simulink model "DynMdlSilver_20171112_1524"  (R2016b)
settings: Solver=VariableStepAuto  StartTime=0.0  StopTime=10.0  RelTol=1e-3
libraries: TM_DynamicModel_Library x117
settings Model: Creator=vpadmaj  LastModifiedBy=vpadmaj

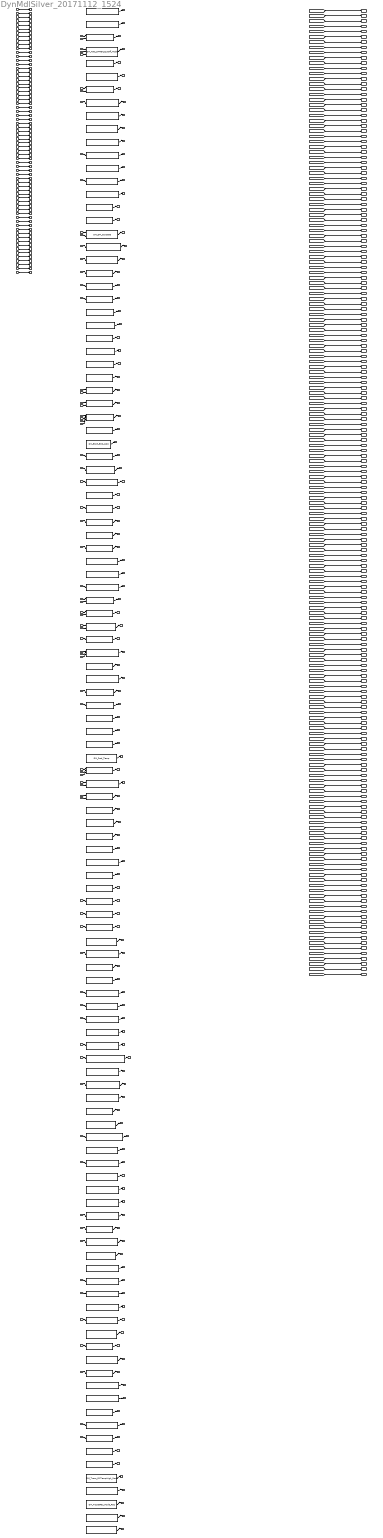
== system DynMdlSilver_20171112_1524 ==
  AAP : Inport
  AAT : Inport  Port=2
  AC_ShutterOpen_Req : Inport  Port=3
  AGB_WaterLevel : Inport  Port=4
  APP : Inport  Port=5
  AirFilOutP_P : Inport  Port=6
  AirFilOutTp_Tp : Inport  Port=7
  AmbAirP_P : Inport  Port=8
  AmbAirTp_Tp : Inport  Port=9
  Bat_Volt : Inport  Port=10
  Bms48_Cur : Inport  Port=11
  Bms48_Tp : Inport  Port=12
  Bms48_Volt : Inport  Port=13
  CacCooltTp_Tp : Inport  Port=14
  CacInTp_Tp : Inport  Port=15
  CacOutTp_Tp : Inport  Port=16
  ClpmpBms_ElecCurrAct : Inport  Port=17
  Dcdc1_CurHvDc : Inport  Port=18
  ECT : Inport  Port=19
  EIS_IgnSwState : Inport  Port=20
  EM2_Curr : Inport  Port=21
  EM2_InvrtTemp : Inport  Port=22
  EM2_Spd : Inport  Port=23
  EM2_Trq : Inport  Port=24
  EM2_TrqPlaus : Inport  Port=25
  EM2_Volt : Inport  Port=26
  ESOC_SOC : Inport  Port=27
  Eac_CurHvDc : Inport  Port=28
  Eac_VoltHvDc : Inport  Port=29
  Em01_CurHvDc : Inport  Port=30
  Em01_TpCooltOutInv : Inport  Port=31
  Em01_VoltHvDc : Inport  Port=32
  Emmo_VoltLinkPN48 : Inport  Port=33
  EngClpmp_FlgOnReq : Inport  Port=34
  EngCoolTp_Tp : Inport  Port=35
  EngCoolTp_TpMdl : Inport  Port=36
  EngOilP_P : Inport  Port=37
  EngOilTp_Tp : Inport  Port=38
  Eng_Fuel_Mass_Flow_Calc : Inport  Port=39
  Eng_Spd : Inport  Port=40
  Eng_Trq : Inport  Port=41
  Eng_Trq_Ind : Inport  Port=42
  ExtAir_Temp_Raw : Inport  Port=43
  Fu_Mp1 : Inport  Port=44
  Gear_State : Inport  Port=45
  IAT : Inport  Port=46
  IMAT : Inport  Port=47
  IntkAir_Temp : Inport  Port=48
  IntkVlvInP_P : Inport  Port=49
  LIN_BpShttrPosReq : Inport  Port=50
  LIN_CF_Spd_Req : Inport  Port=51
  LIN_CP_CACTransSpd_Req : Inport  Port=52
  LIN_RSV_CACTransPos_State : Inport  Port=53
  LIN_ShttrPosReq : Inport  Port=54
  MAF : Inport  Port=55
  Pnct48_DcdcCnvrTemp : Inport  Port=56
  Pnct48_PwrPackCoolOutTemp : Inport  Port=57
  TCM_Oil_Temp : Inport  Port=58
  ThrOutPSnsr_P : Inport  Port=59
  TmBmsCcr_SnsrTp : Inport  Port=60
  TmLtCcr_SnsrTpAct : Inport  Port=61
  TmPmp_EngClpmpLinReqPwm : Inport  Port=62
  Tm_BmsClpmpNReq : Inport  Port=63
  TrbInTp_Tp : Inport  Port=64
  VehMass_Wght_Pred : Inport  Port=65
  Veh_Spd : Inport  Port=66
  n_Eng : Inport  Port=67
  tp_ExhAtExhMnfld : Inport  Port=68
  DM_ACSwOff_Mode : TM_DynamicModel_Library/DM_ACSwOff_Mode
  DM_AC_HtrVlv_Front_Req : TM_DynamicModel_Library/DM_AC_HtrVlv_Front_Req
  DM_AGC_ASSStop_Mode : TM_DynamicModel_Library/DM_AGC_ASSStop_Mode
  DM_AGC_DTREngCutOff_Mode : TM_DynamicModel_Library/DM_AGC_DTREngCutOff_Mode
  DM_AGKInit_Mode : TM_DynamicModel_Library/DM_AGKInit_Mode
  DM_AT2_Mode : TM_DynamicModel_Library/DM_AT2_Mode
  DM_AdapAltitudeTempCorr_Coef : TM_DynamicModel_Library/DM_AdapAltitudeTempCorr_Coef
  DM_AdapAltitude_Coef : TM_DynamicModel_Library/DM_AdapAltitude_Coef
  DM_BMS_Batt_Temp : TM_DynamicModel_Library/DM_BMS_Batt_Temp
  DM_Bat_TotDchaProtnSwtSt : TM_DynamicModel_Library/DM_Bat_TotDchaProtnSwtSt
  DM_ChilExpVlv_RunSt : TM_DynamicModel_Library/DM_ChilExpVlv_RunSt
  DM_ClpmpBms_ElecRpmTrgtAct : TM_DynamicModel_Library/DM_ClpmpBms_ElecRpmTrgtAct
  DM_ClpmpBms_ElecTempAct : TM_DynamicModel_Library/DM_ClpmpBms_ElecTempAct
  DM_ClpmpBms_NAct : TM_DynamicModel_Library/DM_ClpmpBms_NAct
  DM_Cmpr1OutP_P : TM_DynamicModel_Library/DM_Cmpr1OutP_P
  DM_DCDC1_CoolTemp : TM_DynamicModel_Library/DM_DCDC1_CoolTemp
  DM_DCDC1_Temp : TM_DynamicModel_Library/DM_DCDC1_Temp
  DM_DFI_OprState : TM_DynamicModel_Library/DM_DFI_OprState
  DM_DFSO_Mode : TM_DynamicModel_Library/DM_DFSO_Mode
  DM_Dspl_EngShutOff_Time : TM_DynamicModel_Library/DM_Dspl_EngShutOff_Time
  DM_EACHV_Energy_Req : TM_DynamicModel_Library/DM_EACHV_Energy_Req
  DM_EACHV_SwClosed : TM_DynamicModel_Library/DM_EACHV_SwClosed
  DM_EACHV_SwOpen : TM_DynamicModel_Library/DM_EACHV_SwOpen
  DM_EATX_State : TM_DynamicModel_Library/DM_EATX_State
  DM_ECF_Pwr_Req : TM_DynamicModel_Library/DM_ECF_Pwr_Req
  DM_ECOMP_EAC_CompOn_Req : TM_DynamicModel_Library/DM_ECOMP_EAC_CompOn_Req
  DM_ECU_Temp : TM_DynamicModel_Library/DM_ECU_Temp
  DM_EFB_HV_Ready_Mode : TM_DynamicModel_Library/DM_EFB_HV_Ready_Mode
  DM_EM2_Cool_Req : TM_DynamicModel_Library/DM_EM2_Cool_Req
  DM_EM2_StMachn_State : TM_DynamicModel_Library/DM_EM2_StMachn_State
  DM_EM2_State_Req : TM_DynamicModel_Library/DM_EM2_State_Req
  DM_EM2_Temp : TM_DynamicModel_Library/DM_EM2_Temp
  DM_EOBC_Energy_Req : TM_DynamicModel_Library/DM_EOBC_Energy_Req
  DM_ESIG_BMS_SOC : TM_DynamicModel_Library/DM_ESIG_BMS_SOC
  DM_ESIG_BMS_Switch_State : TM_DynamicModel_Library/DM_ESIG_BMS_Switch_State
  DM_ESIG_Dspl_EngShutOff_Time : TM_DynamicModel_Library/DM_ESIG_Dspl_EngShutOff_Time
  DM_Ebtm_FlgHvBatChilCoolReq : TM_DynamicModel_Library/DM_Ebtm_FlgHvBatChilCoolReq
  DM_Ecobc_FlgBatHeatgReq : TM_DynamicModel_Library/DM_Ecobc_FlgBatHeatgReq
  DM_Ecu_St : TM_DynamicModel_Library/DM_Ecu_St
  DM_Ecu_StBusReq : TM_DynamicModel_Library/DM_Ecu_StBusReq
  DM_Efb_FlgHvRdyModPlaus : TM_DynamicModel_Library/DM_Efb_FlgHvRdyModPlaus
  DM_Em_PhaAcCur : TM_DynamicModel_Library/DM_Em_PhaAcCur
  DM_Emm_FlgNetSndrEna : TM_DynamicModel_Library/DM_Emm_FlgNetSndrEna
  DM_EngClpmp_PercPwrReq : TM_DynamicModel_Library/DM_EngClpmp_PercPwrReq
  DM_Eng_Actl_OpMode : TM_DynamicModel_Library/DM_Eng_Actl_OpMode
  DM_Eng_Cyc_Time : TM_DynamicModel_Library/DM_Eng_Cyc_Time
  DM_Eng_RelLoad : TM_DynamicModel_Library/DM_Eng_RelLoad
  DM_Eng_RelLoad_Req : TM_DynamicModel_Library/DM_Eng_RelLoad_Req
  DM_Eng_Run_Mode : TM_DynamicModel_Library/DM_Eng_Run_Mode
  DM_Eng_State_Actl : TM_DynamicModel_Library/DM_Eng_State_Actl
  DM_Eprec_FlgPreCdngAcvMod : TM_DynamicModel_Library/DM_Eprec_FlgPreCdngAcvMod
  DM_Err_ECT_low : TM_DynamicModel_Library/DM_Err_ECT_low
  DM_Esig_BmsTpMax : TM_DynamicModel_Library/DM_Esig_BmsTpMax
  DM_Esig_BmsTpMin : TM_DynamicModel_Library/DM_Esig_BmsTpMin
  DM_Esig_BmsTpTar : TM_DynamicModel_Library/DM_Esig_BmsTpTar
  DM_FRT_Sens : TM_DynamicModel_Library/DM_FRT_Sens
  DM_FirstStrt_Mode : TM_DynamicModel_Library/DM_FirstStrt_Mode
  DM_Fuel_Temp : TM_DynamicModel_Library/DM_Fuel_Temp
  DM_HDC_HybAggr_State : TM_DynamicModel_Library/DM_HDC_HybAggr_State
  DM_HDC_HybSync_State : TM_DynamicModel_Library/DM_HDC_HybSync_State
  DM_HDC_PTReady_Mode : TM_DynamicModel_Library/DM_HDC_PTReady_Mode
  DM_HVAC_CoolVlv_Rq : TM_DynamicModel_Library/DM_HVAC_CoolVlv_Rq
  DM_Hepm_PwrMax48VEcm : TM_DynamicModel_Library/DM_Hepm_PwrMax48VEcm
  DM_Hpmc_StPlgnOpmdDispd : TM_DynamicModel_Library/DM_Hpmc_StPlgnOpmdDispd
  DM_HvacChil_ExpVlvPosnReq : TM_DynamicModel_Library/DM_HvacChil_ExpVlvPosnReq
  DM_Hvac_StDefrstAcv : TM_DynamicModel_Library/DM_Hvac_StDefrstAcv
  DM_IC_Knk_Red_Avg : TM_DynamicModel_Library/DM_IC_Knk_Red_Avg
  DM_IC_Knk_Red_Avg_Actv : TM_DynamicModel_Library/DM_IC_Knk_Red_Avg_Actv
  DM_Idle_Mode_Req : TM_DynamicModel_Library/DM_Idle_Mode_Req
  DM_IgnSwStrtr_Mode : TM_DynamicModel_Library/DM_IgnSwStrtr_Mode
  DM_Ign_Mode : TM_DynamicModel_Library/DM_Ign_Mode
  DM_Injr_Tp : TM_DynamicModel_Library/DM_Injr_Tp
  DM_K15 : TM_DynamicModel_Library/DM_K15
  DM_LIN_BpShttrGrOvrTemp105_Mode : TM_DynamicModel_Library/DM_LIN_BpShttrGrOvrTemp105_Mode
  DM_LIN_BpShttrGrOvrTemp_Mode : TM_DynamicModel_Library/DM_LIN_BpShttrGrOvrTemp_Mode
  DM_LIN_BpShttrPosAct_Val : TM_DynamicModel_Library/DM_LIN_BpShttrPosAct_Val
  DM_LIN_CF_SpdAvg : TM_DynamicModel_Library/DM_LIN_CF_SpdAvg
  DM_LIN_CP_CAC2TransActlSpd : TM_DynamicModel_Library/DM_LIN_CP_CAC2TransActlSpd
  DM_LIN_CP_CAC2TransTp : TM_DynamicModel_Library/DM_LIN_CP_CAC2TransTp
  DM_LIN_CP_CACTransActlSpd : TM_DynamicModel_Library/DM_LIN_CP_CACTransActlSpd
  DM_LIN_CP_CACTransTgtSpd : TM_DynamicModel_Library/DM_LIN_CP_CACTransTgtSpd
  DM_LIN_CP_CACTransTp : TM_DynamicModel_Library/DM_LIN_CP_CACTransTp
  DM_LIN_CP_ECP4TransActlSpd : TM_DynamicModel_Library/DM_LIN_CP_ECP4TransActlSpd
  DM_LIN_CP_ECP4TransTp : TM_DynamicModel_Library/DM_LIN_CP_ECP4TransTp
  DM_LIN_CP_ECP4TransVoltClass : TM_DynamicModel_Library/DM_LIN_CP_ECP4TransVoltClass
  DM_LIN_CP_ECP4TransVoltStat : TM_DynamicModel_Library/DM_LIN_CP_ECP4TransVoltStat
  DM_LIN_RSV1_CACTransPos_State : TM_DynamicModel_Library/DM_LIN_RSV1_CACTransPos_State
  DM_LIN_RSV_CACTransMove_State : TM_DynamicModel_Library/DM_LIN_RSV_CACTransMove_State
  DM_LIN_ShttrPosAct_Val : TM_DynamicModel_Library/DM_LIN_ShttrPosAct_Val
  DM_LIN_ShttrPosMove_State : TM_DynamicModel_Library/DM_LIN_ShttrPosMove_State
  DM_MTX_Mode : TM_DynamicModel_Library/DM_MTX_Mode
  DM_Net_EBoost_CurrCons : TM_DynamicModel_Library/DM_Net_EBoost_CurrCons
  DM_Net_Eboost_PCB_Temp : TM_DynamicModel_Library/DM_Net_Eboost_PCB_Temp
  DM_Odo_Abs_HighRes : TM_DynamicModel_Library/DM_Odo_Abs_HighRes
  DM_Odo_Abs_Long : TM_DynamicModel_Library/DM_Odo_Abs_Long
  DM_Pnct48V_VoltMinThdShutDwnEcm : TM_DynamicModel_Library/DM_Pnct48V_VoltMinThdShutDwnEcm
  DM_Pnct48_HtCoolPwrRq : TM_DynamicModel_Library/DM_Pnct48_HtCoolPwrRq
  DM_Pnct48_PwrPackBatTempMax : TM_DynamicModel_Library/DM_Pnct48_PwrPackBatTempMax
  DM_Pnct48_PwrPackBatTempMin : TM_DynamicModel_Library/DM_Pnct48_PwrPackBatTempMin
  DM_RsvBms_PosnAct : TM_DynamicModel_Library/DM_RsvBms_PosnAct
  DM_RsvLoTpCcr_PosnAvlFlg : TM_DynamicModel_Library/DM_RsvLoTpCcr_PosnAvlFlg
  DM_ScrcmDos_THeatrPmpAftRunReq : TM_DynamicModel_Library/DM_ScrcmDos_THeatrPmpAftRunReq
  DM_TCC_Spd : TM_DynamicModel_Library/DM_TCC_Spd
  DM_Tc_FlgTpCrit : TM_DynamicModel_Library/DM_Tc_FlgTpCrit
  DM_TmBmsCcr_SnsrTpRaw : TM_DynamicModel_Library/DM_TmBmsCcr_SnsrTpRaw
  DM_TmBmsPSnsrChil_VoltRaw : TM_DynamicModel_Library/DM_TmBmsPSnsrChil_VoltRaw
  DM_TmBmsTpSnsrChil_ActVoltRaw : TM_DynamicModel_Library/DM_TmBmsTpSnsrChil_ActVoltRaw
  DM_TmGbOil_PredCtlAcvnFlg : TM_DynamicModel_Library/DM_TmGbOil_PredCtlAcvnFlg
  DM_TmLoTpCcr2_FillLvlVoltRaw : TM_DynamicModel_Library/DM_TmLoTpCcr2_FillLvlVoltRaw
  DM_TmLoTpCcr_SnsrTpRaw : TM_DynamicModel_Library/DM_TmLoTpCcr_SnsrTpRaw
  DM_TmPredHvBatCoolg_TpSpAcvFlg : TM_DynamicModel_Library/DM_TmPredHvBatCoolg_TpSpAcvFlg
  DM_TmPredQckwnsBatCoolt_BatTpSp : TM_DynamicModel_Library/DM_TmPredQckwnsBatCoolt_BatTpSp
  DM_Trans_OilTempHigh_Mode : TM_DynamicModel_Library/DM_Trans_OilTempHigh_Mode
  DM_TrqSetIgn_Mode_Req : TM_DynamicModel_Library/DM_TrqSetIgn_Mode_Req
  DM_TrqSetRes_Mode_Req : TM_DynamicModel_Library/DM_TrqSetRes_Mode_Req
  DM_ag_CamsftExhSp : TM_DynamicModel_Library/DM_ag_CamsftExhSp
  DM_ag_CamsftIntkSp : TM_DynamicModel_Library/DM_ag_CamsftIntkSp
  Dyn_AAP : Outport
  Dyn_AAT : Outport  Port=2
  Dyn_ACSwOff_Mode : Outport  Port=3
  Dyn_AC_HtrVlv_Front_Req : Outport  Port=4
  Dyn_AC_ShutterOpen_Req : Outport  Port=5
  Dyn_AGB_WaterLevel : Outport  Port=6
  Dyn_AGC_ASSStop_Mode : Outport  Port=7
  Dyn_AGC_DTREngCutOff_Mode : Outport  Port=8
  Dyn_AGKInit_Mode : Outport  Port=9
  Dyn_APP : Outport  Port=10
  Dyn_AT2_Mode : Outport  Port=11
  Dyn_AdapAltitudeTempCorr_Coef : Outport  Port=12
  Dyn_AdapAltitude_Coef : Outport  Port=13
  Dyn_AirFilOutP_P : Outport  Port=14
  Dyn_AirFilOutTp_Tp : Outport  Port=15
  Dyn_AmbAirP_P : Outport  Port=16
  Dyn_AmbAirTp_Tp : Outport  Port=17
  Dyn_BMS_Batt_Temp : Outport  Port=18
  Dyn_Bat_TotDchaProtnSwtSt : Outport  Port=19
  Dyn_Bat_Volt : Outport  Port=20
  Dyn_Bms48_Cur : Outport  Port=21
  Dyn_Bms48_Tp : Outport  Port=22
  Dyn_Bms48_Volt : Outport  Port=23
  Dyn_CacCooltTp_Tp : Outport  Port=24
  Dyn_CacInTp_Tp : Outport  Port=25
  Dyn_CacOutTp_Tp : Outport  Port=26
  Dyn_ChilExpVlv_RunSt : Outport  Port=27
  Dyn_ClpmpBms_ElecCurrAct : Outport  Port=28
  Dyn_ClpmpBms_ElecRpmTrgtAct : Outport  Port=29
  Dyn_ClpmpBms_ElecTempAct : Outport  Port=30
  Dyn_ClpmpBms_NAct : Outport  Port=31
  Dyn_Cmpr1OutP_P : Outport  Port=32
  Dyn_DCDC1_CoolTemp : Outport  Port=33
  Dyn_DCDC1_Temp : Outport  Port=34
  Dyn_DFI_OprState : Outport  Port=35
  Dyn_DFSO_Mode : Outport  Port=36
  Dyn_Dcdc1_CurHvDc : Outport  Port=37
  Dyn_Dspl_EngShutOff_Time : Outport  Port=38
  Dyn_EACHV_Energy_Req : Outport  Port=39
  Dyn_EACHV_SwClosed : Outport  Port=40
  Dyn_EACHV_SwOpen : Outport  Port=41
  Dyn_EATX_State : Outport  Port=42
  Dyn_ECF_Pwr_Req : Outport  Port=43
  Dyn_ECOMP_EAC_CompOn_Req : Outport  Port=44
  Dyn_ECT : Outport  Port=45
  Dyn_ECU_Temp : Outport  Port=46
  Dyn_EFB_HV_Ready_Mode : Outport  Port=47
  Dyn_EIS_IgnSwState : Outport  Port=48
  Dyn_EM2_Cool_Req : Outport  Port=49
  Dyn_EM2_Curr : Outport  Port=50
  Dyn_EM2_InvrtTemp : Outport  Port=51
  Dyn_EM2_Spd : Outport  Port=52
  Dyn_EM2_StMachn_State : Outport  Port=53
  Dyn_EM2_State_Req : Outport  Port=54
  Dyn_EM2_Temp : Outport  Port=55
  Dyn_EM2_Trq : Outport  Port=56
  Dyn_EM2_TrqPlaus : Outport  Port=57
  Dyn_EM2_Volt : Outport  Port=58
  Dyn_EOBC_Energy_Req : Outport  Port=59
  Dyn_ESIG_BMS_SOC : Outport  Port=60
  Dyn_ESIG_BMS_Switch_State : Outport  Port=61
  Dyn_ESIG_Dspl_EngShutOff_Time : Outport  Port=62
  Dyn_ESOC_SOC : Outport  Port=63
  Dyn_Eac_CurHvDc : Outport  Port=64
  Dyn_Eac_VoltHvDc : Outport  Port=65
  Dyn_Ebtm_FlgHvBatChilCoolReq : Outport  Port=66
  Dyn_Ecobc_FlgBatHeatgReq : Outport  Port=67
  Dyn_Ecu_St : Outport  Port=68
  Dyn_Ecu_StBusReq : Outport  Port=69
  Dyn_Efb_FlgHvRdyModPlaus : Outport  Port=70
  Dyn_Em01_CurHvDc : Outport  Port=71
  Dyn_Em01_TpCooltOutInv : Outport  Port=72
  Dyn_Em01_VoltHvDc : Outport  Port=73
  Dyn_Em_PhaAcCur : Outport  Port=74
  Dyn_Emm_FlgNetSndrEna : Outport  Port=75
  Dyn_Emmo_VoltLinkPN48 : Outport  Port=76
  Dyn_EngClpmp_FlgOnReq : Outport  Port=77
  Dyn_EngClpmp_PercPwrReq : Outport  Port=78
  Dyn_EngCoolTp_Tp : Outport  Port=79
  Dyn_EngCoolTp_TpMdl : Outport  Port=80
  Dyn_EngOilP_P : Outport  Port=81
  Dyn_EngOilTp_Tp : Outport  Port=82
  Dyn_Eng_Actl_OpMode : Outport  Port=83
  Dyn_Eng_Cyc_Time : Outport  Port=84
  Dyn_Eng_Fuel_Mass_Flow_Calc : Outport  Port=85
  Dyn_Eng_RelLoad : Outport  Port=86
  Dyn_Eng_RelLoad_Req : Outport  Port=87
  Dyn_Eng_Run_Mode : Outport  Port=88
  Dyn_Eng_Spd : Outport  Port=89
  Dyn_Eng_State_Actl : Outport  Port=90
  Dyn_Eng_Trq : Outport  Port=91
  Dyn_Eng_Trq_Ind : Outport  Port=92
  Dyn_Eprec_FlgPreCdngAcvMod : Outport  Port=93
  Dyn_Err_ECT_low : Outport  Port=94
  Dyn_Esig_BmsTpMax : Outport  Port=95
  Dyn_Esig_BmsTpMin : Outport  Port=96
  Dyn_Esig_BmsTpTar : Outport  Port=97
  Dyn_ExtAir_Temp_Raw : Outport  Port=98
  Dyn_FRT_Sens : Outport  Port=99
  Dyn_FirstStrt_Mode : Outport  Port=100
  Dyn_Fu_Mp1 : Outport  Port=101
  Dyn_Fuel_Temp : Outport  Port=102
  Dyn_Gear_State : Outport  Port=103
  Dyn_HDC_HybAggr_State : Outport  Port=104
  Dyn_HDC_HybSync_State : Outport  Port=105
  Dyn_HDC_PTReady_Mode : Outport  Port=106
  Dyn_HVAC_CoolVlv_Rq : Outport  Port=107
  Dyn_Hepm_PwrMax48VEcm : Outport  Port=108
  Dyn_Hpmc_StPlgnOpmdDispd : Outport  Port=109
  Dyn_HvacChil_ExpVlvPosnReq : Outport  Port=110
  Dyn_Hvac_StDefrstAcv : Outport  Port=111
  Dyn_IAT : Outport  Port=112
  Dyn_IC_Knk_Red_Avg : Outport  Port=113
  Dyn_IC_Knk_Red_Avg_Actv : Outport  Port=114
  Dyn_IMAT : Outport  Port=115
  Dyn_Idle_Mode_Req : Outport  Port=116
  Dyn_IgnSwStrtr_Mode : Outport  Port=117
  Dyn_Ign_Mode : Outport  Port=118
  Dyn_Injr_Tp : Outport  Port=119
  Dyn_IntkAir_Temp : Outport  Port=120
  Dyn_IntkVlvInP_P : Outport  Port=121
  Dyn_K15 : Outport  Port=122
  Dyn_LIN_BpShttrGrOvrTemp105_Mode : Outport  Port=123
  Dyn_LIN_BpShttrGrOvrTemp_Mode : Outport  Port=124
  Dyn_LIN_BpShttrPosAct_Val : Outport  Port=125
  Dyn_LIN_BpShttrPosReq : Outport  Port=126
  Dyn_LIN_CF_SpdAvg : Outport  Port=127
  Dyn_LIN_CF_Spd_Req : Outport  Port=128
  Dyn_LIN_CP_CAC2TransActlSpd : Outport  Port=129
  Dyn_LIN_CP_CAC2TransTp : Outport  Port=130
  Dyn_LIN_CP_CACTransActlSpd : Outport  Port=131
  Dyn_LIN_CP_CACTransSpd_Req : Outport  Port=132
  Dyn_LIN_CP_CACTransTgtSpd : Outport  Port=133
  Dyn_LIN_CP_CACTransTp : Outport  Port=134
  Dyn_LIN_CP_ECP4TransActlSpd : Outport  Port=135
  Dyn_LIN_CP_ECP4TransTp : Outport  Port=136
  Dyn_LIN_CP_ECP4TransVoltClass : Outport  Port=137
  Dyn_LIN_CP_ECP4TransVoltStat : Outport  Port=138
  Dyn_LIN_RSV1_CACTransPos_State : Outport  Port=139
  Dyn_LIN_RSV_CACTransMove_State : Outport  Port=140
  Dyn_LIN_RSV_CACTransPos_State : Outport  Port=141
  Dyn_LIN_ShttrPosAct_Val : Outport  Port=142
  Dyn_LIN_ShttrPosMove_State : Outport  Port=143
  Dyn_LIN_ShttrPosReq : Outport  Port=144
  Dyn_MAF : Outport  Port=145
  Dyn_MTX_Mode : Outport  Port=146
  Dyn_Net_EBoost_CurrCons : Outport  Port=147
  Dyn_Net_Eboost_PCB_Temp : Outport  Port=148
  Dyn_Odo_Abs_HighRes : Outport  Port=149
  Dyn_Odo_Abs_Long : Outport  Port=150
  Dyn_Pnct48V_VoltMinThdShutDwnEcm : Outport  Port=151
  Dyn_Pnct48_DcdcCnvrTemp : Outport  Port=152
  Dyn_Pnct48_HtCoolPwrRq : Outport  Port=153
  Dyn_Pnct48_PwrPackBatTempMax : Outport  Port=154
  Dyn_Pnct48_PwrPackBatTempMin : Outport  Port=155
  Dyn_Pnct48_PwrPackCoolOutTemp : Outport  Port=156
  Dyn_RsvBms_PosnAct : Outport  Port=157
  Dyn_RsvLoTpCcr_PosnAvlFlg : Outport  Port=158
  Dyn_ScrcmDos_THeatrPmpAftRunReq : Outport  Port=159
  Dyn_TCC_Spd : Outport  Port=160
  Dyn_TCM_Oil_Temp : Outport  Port=161
  Dyn_Tc_FlgTpCrit : Outport  Port=162
  Dyn_ThrOutPSnsr_P : Outport  Port=163
  Dyn_TmBmsCcr_SnsrTp : Outport  Port=164
  Dyn_TmBmsCcr_SnsrTpRaw : Outport  Port=165
  Dyn_TmBmsPSnsrChil_VoltRaw : Outport  Port=166
  Dyn_TmBmsTpSnsrChil_ActVoltRaw : Outport  Port=167
  Dyn_TmGbOil_PredCtlAcvnFlg : Outport  Port=168
  Dyn_TmLoTpCcr2_FillLvlVoltRaw : Outport  Port=169
  Dyn_TmLoTpCcr_SnsrTpRaw : Outport  Port=170
  Dyn_TmLtCcr_SnsrTpAct : Outport  Port=171
  Dyn_TmPmp_EngClpmpLinReqPwm : Outport  Port=172
  Dyn_TmPredHvBatCoolg_TpSpAcvFlg : Outport  Port=173
  Dyn_TmPredQckwnsBatCoolt_BatTpSp : Outport  Port=174
  Dyn_Tm_BmsClpmpNReq : Outport  Port=175
  Dyn_Trans_OilTempHigh_Mode : Outport  Port=176
  Dyn_TrbInTp_Tp : Outport  Port=177
  Dyn_TrqSetIgn_Mode_Req : Outport  Port=178
  Dyn_TrqSetRes_Mode_Req : Outport  Port=179
  Dyn_VehMass_Wght_Pred : Outport  Port=180
  Dyn_Veh_Spd : Outport  Port=181
  Dyn_ag_CamsftExhSp : Outport  Port=182
  Dyn_ag_CamsftIntkSp : Outport  Port=183
  Dyn_n_Eng : Outport  Port=184
  Dyn_tp_ExhAtExhMnfld : Outport  Port=185
  wires:
  DM_ACSwOff_Mode/1 -> [ACSwOff_Mode]
  DM_AC_HtrVlv_Front_Req/1 -> [AC_HtrVlv_Front_Req]
  [Eng_Spd] -> DM_AGC_ASSStop_Mode/1
  [Eng_Trq] -> DM_AGC_ASSStop_Mode/2
  DM_AGC_ASSStop_Mode/1 -> [AGC_ASSStop_Mode]
  [Eng_Trq] -> DM_AGC_DTREngCutOff_Mode/1
  [EIS_IgnSwState] -> DM_AGC_DTREngCutOff_Mode/2
  [Eng_Spd] -> DM_AGC_DTREngCutOff_Mode/3
  DM_AGC_DTREngCutOff_Mode/1 -> [AGC_DTREngCutOff_Mode]
  DM_AGKInit_Mode/1 -> [AGKInit_Mode]
  DM_AT2_Mode/1 -> [AT2_Mode]
  [AmbAirP_P] -> DM_AdapAltitudeTempCorr_Coef/1
  [IntkAir_Temp] -> DM_AdapAltitudeTempCorr_Coef/2
  DM_AdapAltitudeTempCorr_Coef/1 -> [AdapAltitudeTempCorr_Coef]
  [AmbAirP_P] -> DM_AdapAltitude_Coef/1
  DM_AdapAltitude_Coef/1 -> [AdapAltitude_Coef]
  DM_BMS_Batt_Temp/1 -> [BMS_Batt_Temp]
  DM_Bat_TotDchaProtnSwtSt/1 -> [Bat_TotDchaProtnSwtSt]
  DM_ChilExpVlv_RunSt/1 -> [ChilExpVlv_RunSt]
  [Tm_BmsClpmpNReq] -> DM_ClpmpBms_ElecRpmTrgtAct/1
  DM_ClpmpBms_ElecRpmTrgtAct/1 -> [ClpmpBms_ElecRpmTrgtAct]
  DM_ClpmpBms_ElecTempAct/1 -> [ClpmpBms_ElecTempAct]
  [Tm_BmsClpmpNReq] -> DM_ClpmpBms_NAct/1
  DM_ClpmpBms_NAct/1 -> [ClpmpBms_NAct]
  DM_Cmpr1OutP_P/1 -> [Cmpr1OutP_P]
  DM_DCDC1_CoolTemp/1 -> [DCDC1_CoolTemp]
  DM_DCDC1_Temp/1 -> [DCDC1_Temp]
  [MAF] -> DM_DFI_OprState/1
  [Eng_Fuel_Mass_Flow_Calc] -> DM_DFI_OprState/2
  DM_DFI_OprState/1 -> [DFI_OprState]
  [Veh_Spd] -> DM_DFSO_Mode/1
  DM_DFSO_Mode/1 -> [DFSO_Mode]
  [Eng_Spd] -> DM_Dspl_EngShutOff_Time/1
  DM_Dspl_EngShutOff_Time/1 -> [Dspl_EngShutOff_Time]
  [EIS_IgnSwState] -> DM_EACHV_Energy_Req/1
  DM_EACHV_Energy_Req/1 -> [EACHV_Energy_Req]
  [EIS_IgnSwState] -> DM_EACHV_SwClosed/1
  DM_EACHV_SwClosed/1 -> [EACHV_SwClosed]
  [EIS_IgnSwState] -> DM_EACHV_SwOpen/1
  DM_EACHV_SwOpen/1 -> [EACHV_SwOpen]
  DM_EATX_State/1 -> [EATX_State]
  DM_ECF_Pwr_Req/1 -> [ECF_Pwr_Req]
  DM_ECOMP_EAC_CompOn_Req/1 -> [ECOMP_EAC_CompOn_Req]
  DM_ECU_Temp/1 -> [ECU_Temp]
  DM_EFB_HV_Ready_Mode/1 -> [EFB_HV_Ready_Mode]
  DM_EM2_Cool_Req/1 -> [EM2_Cool_Req]
  [Eng_Spd] -> DM_EM2_StMachn_State/1
  [EIS_IgnSwState] -> DM_EM2_StMachn_State/2
  DM_EM2_StMachn_State/1 -> [EM2_StMachn_State]
  [Eng_Spd] -> DM_EM2_State_Req/1
  [Gear_State] -> DM_EM2_State_Req/2
  DM_EM2_State_Req/1 -> [EM2_State_Req]
  [EM2_Volt] -> DM_EM2_Temp/1
  [EM2_Curr] -> DM_EM2_Temp/2
  [EM2_Trq] -> DM_EM2_Temp/3
  [EM2_Spd] -> DM_EM2_Temp/4
  DM_EM2_Temp/1 -> [EM2_Temp]
  DM_EOBC_Energy_Req/1 -> [EOBC_Energy_Req]
  DM_ESIG_BMS_SOC/1 -> [ESIG_BMS_SOC]
  [EIS_IgnSwState] -> DM_ESIG_BMS_Switch_State/1
  DM_ESIG_BMS_Switch_State/1 -> [ESIG_BMS_Switch_State]
  [Eng_Spd] -> DM_ESIG_Dspl_EngShutOff_Time/1
  DM_ESIG_Dspl_EngShutOff_Time/1 -> [ESIG_Dspl_EngShutOff_Time]
  [Bms48_Tp] -> DM_Ebtm_FlgHvBatChilCoolReq/1
  DM_Ebtm_FlgHvBatChilCoolReq/1 -> [Ebtm_FlgHvBatChilCoolReq]
  DM_Ecobc_FlgBatHeatgReq/1 -> [Ecobc_FlgBatHeatgReq]
  [EIS_IgnSwState] -> DM_Ecu_St/1
  DM_Ecu_St/1 -> [Ecu_St]
  [EIS_IgnSwState] -> DM_Ecu_StBusReq/1
  DM_Ecu_StBusReq/1 -> [Ecu_StBusReq]
  DM_Efb_FlgHvRdyModPlaus/1 -> [Efb_FlgHvRdyModPlaus]
  [EM2_Trq] -> DM_Em_PhaAcCur/1
  DM_Em_PhaAcCur/1 -> [Em_PhaAcCur]
  DM_Emm_FlgNetSndrEna/1 -> [Emm_FlgNetSndrEna]
  DM_EngClpmp_PercPwrReq/1 -> [EngClpmp_PercPwrReq]
  [Eng_State_Actl] -> DM_Eng_Actl_OpMode/1
  DM_Eng_Actl_OpMode/1 -> [Eng_Actl_OpMode]
  [Eng_Spd] -> DM_Eng_Cyc_Time/1
  [EIS_IgnSwState] -> DM_Eng_Cyc_Time/2
  DM_Eng_Cyc_Time/1 -> [Eng_Cyc_Time]
  [MAF] -> DM_Eng_RelLoad/1
  [Eng_Spd] -> DM_Eng_RelLoad/2
  DM_Eng_RelLoad/1 -> [Eng_RelLoad]
  [MAF] -> DM_Eng_RelLoad_Req/1
  [Eng_Spd] -> DM_Eng_RelLoad_Req/2
  DM_Eng_RelLoad_Req/1 -> [Eng_RelLoad_Req]
  [Eng_Spd] -> DM_Eng_Run_Mode/1
  DM_Eng_Run_Mode/1 -> [Eng_Run_Mode]
  [K15] -> DM_Eng_State_Actl/1
  [Eng_Spd] -> DM_Eng_State_Actl/2
  [AGC_ASSStop_Mode] -> DM_Eng_State_Actl/3
  DM_Eng_State_Actl/1 -> [Eng_State_Actl]
  DM_Eprec_FlgPreCdngAcvMod/1 -> [Eprec_FlgPreCdngAcvMod]
  DM_Err_ECT_low/1 -> [Err_ECT_low]
  [Bms48_Tp] -> DM_Esig_BmsTpMax/1
  DM_Esig_BmsTpMax/1 -> [Esig_BmsTpMax]
  [Bms48_Tp] -> DM_Esig_BmsTpMin/1
  DM_Esig_BmsTpMin/1 -> [Esig_BmsTpMin]
  DM_Esig_BmsTpTar/1 -> [Esig_BmsTpTar]
  DM_FRT_Sens/1 -> [FRT_Sens]
  DM_FirstStrt_Mode/1 -> [FirstStrt_Mode]
  DM_Fuel_Temp/1 -> [Fuel_Temp]
  [EIS_IgnSwState] -> DM_HDC_HybAggr_State/1
  [Eng_Spd] -> DM_HDC_HybAggr_State/2
  [Gear_State] -> DM_HDC_HybAggr_State/3
  DM_HDC_HybAggr_State/1 -> [HDC_HybAggr_State]
  [Eng_Spd] -> DM_HDC_HybSync_State/1
  [Eng_Trq] -> DM_HDC_HybSync_State/2
  DM_HDC_HybSync_State/1 -> [HDC_HybSync_State]
  [Eng_Spd] -> DM_HDC_PTReady_Mode/1
  [EIS_IgnSwState] -> DM_HDC_PTReady_Mode/2
  DM_HDC_PTReady_Mode/1 -> [HDC_PTReady_Mode]
  DM_HVAC_CoolVlv_Rq/1 -> [HVAC_CoolVlv_Rq]
  DM_Hepm_PwrMax48VEcm/1 -> [Hepm_PwrMax48VEcm]
  DM_Hpmc_StPlgnOpmdDispd/1 -> [Hpmc_StPlgnOpmdDispd]
  DM_HvacChil_ExpVlvPosnReq/1 -> [HvacChil_ExpVlvPosnReq]
  DM_Hvac_StDefrstAcv/1 -> [Hvac_StDefrstAcv]
  DM_IC_Knk_Red_Avg/1 -> [IC_Knk_Red_Avg]
  DM_IC_Knk_Red_Avg_Actv/1 -> [IC_Knk_Red_Avg_Actv]
  [APP] -> DM_Idle_Mode_Req/1
  DM_Idle_Mode_Req/1 -> [Idle_Mode_Req]
  [EIS_IgnSwState] -> DM_IgnSwStrtr_Mode/1
  DM_IgnSwStrtr_Mode/1 -> [IgnSwStrtr_Mode]
  [EIS_IgnSwState] -> DM_Ign_Mode/1
  DM_Ign_Mode/1 -> [Ign_Mode]
  DM_Injr_Tp/1 -> [Injr_Tp]
  [EIS_IgnSwState] -> DM_K15/1
  DM_K15/1 -> [K15]
  DM_LIN_BpShttrGrOvrTemp105_Mode/1 -> [LIN_BpShttrGrOvrTemp105_Mode]
  DM_LIN_BpShttrGrOvrTemp_Mode/1 -> [LIN_BpShttrGrOvrTemp_Mode]
  [LIN_BpShttrPosReq] -> DM_LIN_BpShttrPosAct_Val/1
  DM_LIN_BpShttrPosAct_Val/1 -> [LIN_BpShttrPosAct_Val]
  [LIN_CF_Spd_Req] -> DM_LIN_CF_SpdAvg/1
  DM_LIN_CF_SpdAvg/1 -> [LIN_CF_SpdAvg]
  [Tm_BmsClpmpNReq] -> DM_LIN_CP_CAC2TransActlSpd/1
  DM_LIN_CP_CAC2TransActlSpd/1 -> [LIN_CP_CAC2TransActlSpd]
  DM_LIN_CP_CAC2TransTp/1 -> [LIN_CP_CAC2TransTp]
  [LIN_CP_CACTransSpd_Req] -> DM_LIN_CP_CACTransActlSpd/1
  DM_LIN_CP_CACTransActlSpd/1 -> [LIN_CP_CACTransActlSpd]
  [LIN_CP_CACTransSpd_Req] -> DM_LIN_CP_CACTransTgtSpd/1
  DM_LIN_CP_CACTransTgtSpd/1 -> [LIN_CP_CACTransTgtSpd]
  DM_LIN_CP_CACTransTp/1 -> [LIN_CP_CACTransTp]
  [TmPmp_EngClpmpLinReqPwm] -> DM_LIN_CP_ECP4TransActlSpd/1
  DM_LIN_CP_ECP4TransActlSpd/1 -> [LIN_CP_ECP4TransActlSpd]
  DM_LIN_CP_ECP4TransTp/1 -> [LIN_CP_ECP4TransTp]
  DM_LIN_CP_ECP4TransVoltClass/1 -> [LIN_CP_ECP4TransVoltClass]
  DM_LIN_CP_ECP4TransVoltStat/1 -> [LIN_CP_ECP4TransVoltStat]
  [LIN_RSV_CACTransPos_State] -> DM_LIN_RSV1_CACTransPos_State/1
  DM_LIN_RSV1_CACTransPos_State/1 -> [LIN_RSV1_CACTransPos_State]
  DM_LIN_RSV_CACTransMove_State/1 -> [LIN_RSV_CACTransMove_State]
  [LIN_ShttrPosReq] -> DM_LIN_ShttrPosAct_Val/1
  DM_LIN_ShttrPosAct_Val/1 -> [LIN_ShttrPosAct_Val]
  DM_LIN_ShttrPosMove_State/1 -> [LIN_ShttrPosMove_State]
  DM_MTX_Mode/1 -> [MTX_Mode]
  DM_Net_EBoost_CurrCons/1 -> [Net_EBoost_CurrCons]
  [CacInTp_Tp] -> DM_Net_Eboost_PCB_Temp/1
  DM_Net_Eboost_PCB_Temp/1 -> [Net_Eboost_PCB_Temp]
  [Veh_Spd] -> DM_Odo_Abs_HighRes/1
  DM_Odo_Abs_HighRes/1 -> [Odo_Abs_HighRes]
  [Veh_Spd] -> DM_Odo_Abs_Long/1
  DM_Odo_Abs_Long/1 -> [Odo_Abs_Long]
  DM_Pnct48V_VoltMinThdShutDwnEcm/1 -> [Pnct48V_VoltMinThdShutDwnEcm]
  DM_Pnct48_HtCoolPwrRq/1 -> [Pnct48_HtCoolPwrRq]
  [Bms48_Tp] -> DM_Pnct48_PwrPackBatTempMax/1
  DM_Pnct48_PwrPackBatTempMax/1 -> [Pnct48_PwrPackBatTempMax]
  [Bms48_Tp] -> DM_Pnct48_PwrPackBatTempMin/1
  DM_Pnct48_PwrPackBatTempMin/1 -> [Pnct48_PwrPackBatTempMin]
  DM_RsvBms_PosnAct/1 -> [RsvBms_PosnAct]
  [LIN_RSV_CACTransPos_State] -> DM_RsvLoTpCcr_PosnAvlFlg/1
  DM_RsvLoTpCcr_PosnAvlFlg/1 -> [RsvLoTpCcr_PosnAvlFlg]
  DM_ScrcmDos_THeatrPmpAftRunReq/1 -> [ScrcmDos_THeatrPmpAftRunReq]
  [Eng_Spd] -> DM_TCC_Spd/1
  DM_TCC_Spd/1 -> [TCC_Spd]
  DM_Tc_FlgTpCrit/1 -> [Tc_FlgTpCrit]
  [TmBmsCcr_SnsrTp] -> DM_TmBmsCcr_SnsrTpRaw/1
  DM_TmBmsCcr_SnsrTpRaw/1 -> [TmBmsCcr_SnsrTpRaw]
  DM_TmBmsPSnsrChil_VoltRaw/1 -> [TmBmsPSnsrChil_VoltRaw]
  DM_TmBmsTpSnsrChil_ActVoltRaw/1 -> [TmBmsTpSnsrChil_ActVoltRaw]
  DM_TmGbOil_PredCtlAcvnFlg/1 -> [TmGbOil_PredCtlAcvnFlg]
  [AGB_WaterLevel] -> DM_TmLoTpCcr2_FillLvlVoltRaw/1
  DM_TmLoTpCcr2_FillLvlVoltRaw/1 -> [TmLoTpCcr2_FillLvlVoltRaw]
  [TmLtCcr_SnsrTpAct] -> DM_TmLoTpCcr_SnsrTpRaw/1
  DM_TmLoTpCcr_SnsrTpRaw/1 -> [TmLoTpCcr_SnsrTpRaw]
  DM_TmPredHvBatCoolg_TpSpAcvFlg/1 -> [TmPredHvBatCoolg_TpSpAcvFlg]
  DM_TmPredQckwnsBatCoolt_BatTpSp/1 -> [TmPredQckwnsBatCoolt_BatTpSp]
  DM_Trans_OilTempHigh_Mode/1 -> [Trans_OilTempHigh_Mode]
  DM_TrqSetIgn_Mode_Req/1 -> [TrqSetIgn_Mode_Req]
  DM_TrqSetRes_Mode_Req/1 -> [TrqSetRes_Mode_Req]
  DM_ag_CamsftExhSp/1 -> [ag_CamsftExhSp]
  DM_ag_CamsftIntkSp/1 -> [ag_CamsftIntkSp]
  AAP/1 -> [AAP]
  AAT/1 -> [AAT]
  AC_ShutterOpen_Req/1 -> [AC_ShutterOpen_Req]
  AGB_WaterLevel/1 -> [AGB_WaterLevel]
  APP/1 -> [APP]
  AirFilOutP_P/1 -> [AirFilOutP_P]
  AirFilOutTp_Tp/1 -> [AirFilOutTp_Tp]
  AmbAirP_P/1 -> [AmbAirP_P]
  AmbAirTp_Tp/1 -> [AmbAirTp_Tp]
  Bat_Volt/1 -> [Bat_Volt]
  Bms48_Cur/1 -> [Bms48_Cur]
  Bms48_Tp/1 -> [Bms48_Tp]
  Bms48_Volt/1 -> [Bms48_Volt]
  CacCooltTp_Tp/1 -> [CacCooltTp_Tp]
  CacInTp_Tp/1 -> [CacInTp_Tp]
  CacOutTp_Tp/1 -> [CacOutTp_Tp]
  ClpmpBms_ElecCurrAct/1 -> [ClpmpBms_ElecCurrAct]
  Dcdc1_CurHvDc/1 -> [Dcdc1_CurHvDc]
  ECT/1 -> [ECT]
  EIS_IgnSwState/1 -> [EIS_IgnSwState]
  EM2_Curr/1 -> [EM2_Curr]
  EM2_InvrtTemp/1 -> [EM2_InvrtTemp]
  EM2_Spd/1 -> [EM2_Spd]
  EM2_Trq/1 -> [EM2_Trq]
  EM2_TrqPlaus/1 -> [EM2_TrqPlaus]
  EM2_Volt/1 -> [EM2_Volt]
  ESOC_SOC/1 -> [ESOC_SOC]
  Eac_CurHvDc/1 -> [Eac_CurHvDc]
  Eac_VoltHvDc/1 -> [Eac_VoltHvDc]
  Em01_CurHvDc/1 -> [Em01_CurHvDc]
  Em01_TpCooltOutInv/1 -> [Em01_TpCooltOutInv]
  Em01_VoltHvDc/1 -> [Em01_VoltHvDc]
  Emmo_VoltLinkPN48/1 -> [Emmo_VoltLinkPN48]
  EngClpmp_FlgOnReq/1 -> [EngClpmp_FlgOnReq]
  EngCoolTp_Tp/1 -> [EngCoolTp_Tp]
  EngCoolTp_TpMdl/1 -> [EngCoolTp_TpMdl]
  EngOilP_P/1 -> [EngOilP_P]
  EngOilTp_Tp/1 -> [EngOilTp_Tp]
  Eng_Fuel_Mass_Flow_Calc/1 -> [Eng_Fuel_Mass_Flow_Calc]
  Eng_Spd/1 -> [Eng_Spd]
  Eng_Trq/1 -> [Eng_Trq]
  Eng_Trq_Ind/1 -> [Eng_Trq_Ind]
  ExtAir_Temp_Raw/1 -> [ExtAir_Temp_Raw]
  Fu_Mp1/1 -> [Fu_Mp1]
  Gear_State/1 -> [Gear_State]
  IAT/1 -> [IAT]
  IMAT/1 -> [IMAT]
  IntkAir_Temp/1 -> [IntkAir_Temp]
  IntkVlvInP_P/1 -> [IntkVlvInP_P]
  LIN_BpShttrPosReq/1 -> [LIN_BpShttrPosReq]
  LIN_CF_Spd_Req/1 -> [LIN_CF_Spd_Req]
  LIN_CP_CACTransSpd_Req/1 -> [LIN_CP_CACTransSpd_Req]
  LIN_RSV_CACTransPos_State/1 -> [LIN_RSV_CACTransPos_State]
  LIN_ShttrPosReq/1 -> [LIN_ShttrPosReq]
  MAF/1 -> [MAF]
  Pnct48_DcdcCnvrTemp/1 -> [Pnct48_DcdcCnvrTemp]
  Pnct48_PwrPackCoolOutTemp/1 -> [Pnct48_PwrPackCoolOutTemp]
  TCM_Oil_Temp/1 -> [TCM_Oil_Temp]
  ThrOutPSnsr_P/1 -> [ThrOutPSnsr_P]
  TmBmsCcr_SnsrTp/1 -> [TmBmsCcr_SnsrTp]
  TmLtCcr_SnsrTpAct/1 -> [TmLtCcr_SnsrTpAct]
  TmPmp_EngClpmpLinReqPwm/1 -> [TmPmp_EngClpmpLinReqPwm]
  Tm_BmsClpmpNReq/1 -> [Tm_BmsClpmpNReq]
  TrbInTp_Tp/1 -> [TrbInTp_Tp]
  VehMass_Wght_Pred/1 -> [VehMass_Wght_Pred]
  Veh_Spd/1 -> [Veh_Spd]
  n_Eng/1 -> [n_Eng]
  tp_ExhAtExhMnfld/1 -> [tp_ExhAtExhMnfld]
  [AAP] -> Dyn_AAP/1
  [AAT] -> Dyn_AAT/1
  [ACSwOff_Mode] -> Dyn_ACSwOff_Mode/1
  [AC_HtrVlv_Front_Req] -> Dyn_AC_HtrVlv_Front_Req/1
  [AC_ShutterOpen_Req] -> Dyn_AC_ShutterOpen_Req/1
  [AGB_WaterLevel] -> Dyn_AGB_WaterLevel/1
  [AGC_ASSStop_Mode] -> Dyn_AGC_ASSStop_Mode/1
  [AGC_DTREngCutOff_Mode] -> Dyn_AGC_DTREngCutOff_Mode/1
  [AGKInit_Mode] -> Dyn_AGKInit_Mode/1
  [APP] -> Dyn_APP/1
  [AT2_Mode] -> Dyn_AT2_Mode/1
  [AdapAltitudeTempCorr_Coef] -> Dyn_AdapAltitudeTempCorr_Coef/1
  [AdapAltitude_Coef] -> Dyn_AdapAltitude_Coef/1
  [AirFilOutP_P] -> Dyn_AirFilOutP_P/1
  [AirFilOutTp_Tp] -> Dyn_AirFilOutTp_Tp/1
  [AmbAirP_P] -> Dyn_AmbAirP_P/1
  [AmbAirTp_Tp] -> Dyn_AmbAirTp_Tp/1
  [BMS_Batt_Temp] -> Dyn_BMS_Batt_Temp/1
  [Bat_TotDchaProtnSwtSt] -> Dyn_Bat_TotDchaProtnSwtSt/1
  [Bat_Volt] -> Dyn_Bat_Volt/1
  [Bms48_Cur] -> Dyn_Bms48_Cur/1
  [Bms48_Tp] -> Dyn_Bms48_Tp/1
  [Bms48_Volt] -> Dyn_Bms48_Volt/1
  [CacCooltTp_Tp] -> Dyn_CacCooltTp_Tp/1
  [CacInTp_Tp] -> Dyn_CacInTp_Tp/1
  [CacOutTp_Tp] -> Dyn_CacOutTp_Tp/1
  [ChilExpVlv_RunSt] -> Dyn_ChilExpVlv_RunSt/1
  [ClpmpBms_ElecCurrAct] -> Dyn_ClpmpBms_ElecCurrAct/1
  [ClpmpBms_ElecRpmTrgtAct] -> Dyn_ClpmpBms_ElecRpmTrgtAct/1
  [ClpmpBms_ElecTempAct] -> Dyn_ClpmpBms_ElecTempAct/1
  [ClpmpBms_NAct] -> Dyn_ClpmpBms_NAct/1
  [Cmpr1OutP_P] -> Dyn_Cmpr1OutP_P/1
  [DCDC1_CoolTemp] -> Dyn_DCDC1_CoolTemp/1
  [DCDC1_Temp] -> Dyn_DCDC1_Temp/1
  [DFI_OprState] -> Dyn_DFI_OprState/1
  [DFSO_Mode] -> Dyn_DFSO_Mode/1
  [Dcdc1_CurHvDc] -> Dyn_Dcdc1_CurHvDc/1
  [Dspl_EngShutOff_Time] -> Dyn_Dspl_EngShutOff_Time/1
  [EACHV_Energy_Req] -> Dyn_EACHV_Energy_Req/1
  [EACHV_SwClosed] -> Dyn_EACHV_SwClosed/1
  [EACHV_SwOpen] -> Dyn_EACHV_SwOpen/1
  [EATX_State] -> Dyn_EATX_State/1
  [ECF_Pwr_Req] -> Dyn_ECF_Pwr_Req/1
  [ECOMP_EAC_CompOn_Req] -> Dyn_ECOMP_EAC_CompOn_Req/1
  [ECT] -> Dyn_ECT/1
  [ECU_Temp] -> Dyn_ECU_Temp/1
  [EFB_HV_Ready_Mode] -> Dyn_EFB_HV_Ready_Mode/1
  [EIS_IgnSwState] -> Dyn_EIS_IgnSwState/1
  [EM2_Cool_Req] -> Dyn_EM2_Cool_Req/1
  [EM2_Curr] -> Dyn_EM2_Curr/1
  [EM2_InvrtTemp] -> Dyn_EM2_InvrtTemp/1
  [EM2_Spd] -> Dyn_EM2_Spd/1
  [EM2_StMachn_State] -> Dyn_EM2_StMachn_State/1
  [EM2_State_Req] -> Dyn_EM2_State_Req/1
  [EM2_Temp] -> Dyn_EM2_Temp/1
  [EM2_Trq] -> Dyn_EM2_Trq/1
  [EM2_TrqPlaus] -> Dyn_EM2_TrqPlaus/1
  [EM2_Volt] -> Dyn_EM2_Volt/1
  [EOBC_Energy_Req] -> Dyn_EOBC_Energy_Req/1
  [ESIG_BMS_SOC] -> Dyn_ESIG_BMS_SOC/1
  [ESIG_BMS_Switch_State] -> Dyn_ESIG_BMS_Switch_State/1
  [ESIG_Dspl_EngShutOff_Time] -> Dyn_ESIG_Dspl_EngShutOff_Time/1
  [ESOC_SOC] -> Dyn_ESOC_SOC/1
  [Eac_CurHvDc] -> Dyn_Eac_CurHvDc/1
  [Eac_VoltHvDc] -> Dyn_Eac_VoltHvDc/1
  [Ebtm_FlgHvBatChilCoolReq] -> Dyn_Ebtm_FlgHvBatChilCoolReq/1
  [Ecobc_FlgBatHeatgReq] -> Dyn_Ecobc_FlgBatHeatgReq/1
  [Ecu_St] -> Dyn_Ecu_St/1
  [Ecu_StBusReq] -> Dyn_Ecu_StBusReq/1
  [Efb_FlgHvRdyModPlaus] -> Dyn_Efb_FlgHvRdyModPlaus/1
  [Em01_CurHvDc] -> Dyn_Em01_CurHvDc/1
  [Em01_TpCooltOutInv] -> Dyn_Em01_TpCooltOutInv/1
  [Em01_VoltHvDc] -> Dyn_Em01_VoltHvDc/1
  [Em_PhaAcCur] -> Dyn_Em_PhaAcCur/1
  [Emm_FlgNetSndrEna] -> Dyn_Emm_FlgNetSndrEna/1
  [Emmo_VoltLinkPN48] -> Dyn_Emmo_VoltLinkPN48/1
  [EngClpmp_FlgOnReq] -> Dyn_EngClpmp_FlgOnReq/1
  [EngClpmp_PercPwrReq] -> Dyn_EngClpmp_PercPwrReq/1
  [EngCoolTp_Tp] -> Dyn_EngCoolTp_Tp/1
  [EngCoolTp_TpMdl] -> Dyn_EngCoolTp_TpMdl/1
  [EngOilP_P] -> Dyn_EngOilP_P/1
  [EngOilTp_Tp] -> Dyn_EngOilTp_Tp/1
  [Eng_Actl_OpMode] -> Dyn_Eng_Actl_OpMode/1
  [Eng_Cyc_Time] -> Dyn_Eng_Cyc_Time/1
  [Eng_Fuel_Mass_Flow_Calc] -> Dyn_Eng_Fuel_Mass_Flow_Calc/1
  [Eng_RelLoad] -> Dyn_Eng_RelLoad/1
  [Eng_RelLoad_Req] -> Dyn_Eng_RelLoad_Req/1
  [Eng_Run_Mode] -> Dyn_Eng_Run_Mode/1
  [Eng_Spd] -> Dyn_Eng_Spd/1
  [Eng_State_Actl] -> Dyn_Eng_State_Actl/1
  [Eng_Trq] -> Dyn_Eng_Trq/1
  [Eng_Trq_Ind] -> Dyn_Eng_Trq_Ind/1
  [Eprec_FlgPreCdngAcvMod] -> Dyn_Eprec_FlgPreCdngAcvMod/1
  [Err_ECT_low] -> Dyn_Err_ECT_low/1
  [Esig_BmsTpMax] -> Dyn_Esig_BmsTpMax/1
  [Esig_BmsTpMin] -> Dyn_Esig_BmsTpMin/1
  [Esig_BmsTpTar] -> Dyn_Esig_BmsTpTar/1
  [ExtAir_Temp_Raw] -> Dyn_ExtAir_Temp_Raw/1
  [FRT_Sens] -> Dyn_FRT_Sens/1
  [FirstStrt_Mode] -> Dyn_FirstStrt_Mode/1
  [Fu_Mp1] -> Dyn_Fu_Mp1/1
  [Fuel_Temp] -> Dyn_Fuel_Temp/1
  [Gear_State] -> Dyn_Gear_State/1
  [HDC_HybAggr_State] -> Dyn_HDC_HybAggr_State/1
  [HDC_HybSync_State] -> Dyn_HDC_HybSync_State/1
  [HDC_PTReady_Mode] -> Dyn_HDC_PTReady_Mode/1
  [HVAC_CoolVlv_Rq] -> Dyn_HVAC_CoolVlv_Rq/1
  [Hepm_PwrMax48VEcm] -> Dyn_Hepm_PwrMax48VEcm/1
  [Hpmc_StPlgnOpmdDispd] -> Dyn_Hpmc_StPlgnOpmdDispd/1
  [HvacChil_ExpVlvPosnReq] -> Dyn_HvacChil_ExpVlvPosnReq/1
  [Hvac_StDefrstAcv] -> Dyn_Hvac_StDefrstAcv/1
  [IAT] -> Dyn_IAT/1
  [IC_Knk_Red_Avg] -> Dyn_IC_Knk_Red_Avg/1
  [IC_Knk_Red_Avg_Actv] -> Dyn_IC_Knk_Red_Avg_Actv/1
  [IMAT] -> Dyn_IMAT/1
  [Idle_Mode_Req] -> Dyn_Idle_Mode_Req/1
  [IgnSwStrtr_Mode] -> Dyn_IgnSwStrtr_Mode/1
  [Ign_Mode] -> Dyn_Ign_Mode/1
  [Injr_Tp] -> Dyn_Injr_Tp/1
  [IntkAir_Temp] -> Dyn_IntkAir_Temp/1
  [IntkVlvInP_P] -> Dyn_IntkVlvInP_P/1
  [K15] -> Dyn_K15/1
  [LIN_BpShttrGrOvrTemp105_Mode] -> Dyn_LIN_BpShttrGrOvrTemp105_Mode/1
  [LIN_BpShttrGrOvrTemp_Mode] -> Dyn_LIN_BpShttrGrOvrTemp_Mode/1
  [LIN_BpShttrPosAct_Val] -> Dyn_LIN_BpShttrPosAct_Val/1
  [LIN_BpShttrPosReq] -> Dyn_LIN_BpShttrPosReq/1
  [LIN_CF_SpdAvg] -> Dyn_LIN_CF_SpdAvg/1
  [LIN_CF_Spd_Req] -> Dyn_LIN_CF_Spd_Req/1
  [LIN_CP_CAC2TransActlSpd] -> Dyn_LIN_CP_CAC2TransActlSpd/1
  [LIN_CP_CAC2TransTp] -> Dyn_LIN_CP_CAC2TransTp/1
  [LIN_CP_CACTransActlSpd] -> Dyn_LIN_CP_CACTransActlSpd/1
  [LIN_CP_CACTransSpd_Req] -> Dyn_LIN_CP_CACTransSpd_Req/1
  [LIN_CP_CACTransTgtSpd] -> Dyn_LIN_CP_CACTransTgtSpd/1
  [LIN_CP_CACTransTp] -> Dyn_LIN_CP_CACTransTp/1
  [LIN_CP_ECP4TransActlSpd] -> Dyn_LIN_CP_ECP4TransActlSpd/1
  [LIN_CP_ECP4TransTp] -> Dyn_LIN_CP_ECP4TransTp/1
  [LIN_CP_ECP4TransVoltClass] -> Dyn_LIN_CP_ECP4TransVoltClass/1
  [LIN_CP_ECP4TransVoltStat] -> Dyn_LIN_CP_ECP4TransVoltStat/1
  [LIN_RSV1_CACTransPos_State] -> Dyn_LIN_RSV1_CACTransPos_State/1
  [LIN_RSV_CACTransMove_State] -> Dyn_LIN_RSV_CACTransMove_State/1
  [LIN_RSV_CACTransPos_State] -> Dyn_LIN_RSV_CACTransPos_State/1
  [LIN_ShttrPosAct_Val] -> Dyn_LIN_ShttrPosAct_Val/1
  [LIN_ShttrPosMove_State] -> Dyn_LIN_ShttrPosMove_State/1
  [LIN_ShttrPosReq] -> Dyn_LIN_ShttrPosReq/1
  [MAF] -> Dyn_MAF/1
  [MTX_Mode] -> Dyn_MTX_Mode/1
  [Net_EBoost_CurrCons] -> Dyn_Net_EBoost_CurrCons/1
  [Net_Eboost_PCB_Temp] -> Dyn_Net_Eboost_PCB_Temp/1
  [Odo_Abs_HighRes] -> Dyn_Odo_Abs_HighRes/1
  [Odo_Abs_Long] -> Dyn_Odo_Abs_Long/1
  [Pnct48V_VoltMinThdShutDwnEcm] -> Dyn_Pnct48V_VoltMinThdShutDwnEcm/1
  [Pnct48_DcdcCnvrTemp] -> Dyn_Pnct48_DcdcCnvrTemp/1
  [Pnct48_HtCoolPwrRq] -> Dyn_Pnct48_HtCoolPwrRq/1
  [Pnct48_PwrPackBatTempMax] -> Dyn_Pnct48_PwrPackBatTempMax/1
  [Pnct48_PwrPackBatTempMin] -> Dyn_Pnct48_PwrPackBatTempMin/1
  [Pnct48_PwrPackCoolOutTemp] -> Dyn_Pnct48_PwrPackCoolOutTemp/1
  [RsvBms_PosnAct] -> Dyn_RsvBms_PosnAct/1
  [RsvLoTpCcr_PosnAvlFlg] -> Dyn_RsvLoTpCcr_PosnAvlFlg/1
  [ScrcmDos_THeatrPmpAftRunReq] -> Dyn_ScrcmDos_THeatrPmpAftRunReq/1
  [TCC_Spd] -> Dyn_TCC_Spd/1
  [TCM_Oil_Temp] -> Dyn_TCM_Oil_Temp/1
  [Tc_FlgTpCrit] -> Dyn_Tc_FlgTpCrit/1
  [ThrOutPSnsr_P] -> Dyn_ThrOutPSnsr_P/1
  [TmBmsCcr_SnsrTp] -> Dyn_TmBmsCcr_SnsrTp/1
  [TmBmsCcr_SnsrTpRaw] -> Dyn_TmBmsCcr_SnsrTpRaw/1
  [TmBmsPSnsrChil_VoltRaw] -> Dyn_TmBmsPSnsrChil_VoltRaw/1
  [TmBmsTpSnsrChil_ActVoltRaw] -> Dyn_TmBmsTpSnsrChil_ActVoltRaw/1
  [TmGbOil_PredCtlAcvnFlg] -> Dyn_TmGbOil_PredCtlAcvnFlg/1
  [TmLoTpCcr2_FillLvlVoltRaw] -> Dyn_TmLoTpCcr2_FillLvlVoltRaw/1
  [TmLoTpCcr_SnsrTpRaw] -> Dyn_TmLoTpCcr_SnsrTpRaw/1
  [TmLtCcr_SnsrTpAct] -> Dyn_TmLtCcr_SnsrTpAct/1
  [TmPmp_EngClpmpLinReqPwm] -> Dyn_TmPmp_EngClpmpLinReqPwm/1
  [TmPredHvBatCoolg_TpSpAcvFlg] -> Dyn_TmPredHvBatCoolg_TpSpAcvFlg/1
  [TmPredQckwnsBatCoolt_BatTpSp] -> Dyn_TmPredQckwnsBatCoolt_BatTpSp/1
  [Tm_BmsClpmpNReq] -> Dyn_Tm_BmsClpmpNReq/1
  [Trans_OilTempHigh_Mode] -> Dyn_Trans_OilTempHigh_Mode/1
  [TrbInTp_Tp] -> Dyn_TrbInTp_Tp/1
  [TrqSetIgn_Mode_Req] -> Dyn_TrqSetIgn_Mode_Req/1
  [TrqSetRes_Mode_Req] -> Dyn_TrqSetRes_Mode_Req/1
  [VehMass_Wght_Pred] -> Dyn_VehMass_Wght_Pred/1
  [Veh_Spd] -> Dyn_Veh_Spd/1
  [ag_CamsftExhSp] -> Dyn_ag_CamsftExhSp/1
  [ag_CamsftIntkSp] -> Dyn_ag_CamsftIntkSp/1
  [n_Eng] -> Dyn_n_Eng/1
  [tp_ExhAtExhMnfld] -> Dyn_tp_ExhAtExhMnfld/1
